simulink model "example2"  (R2013b)
settings: Solver=ode3  StartTime=0.0  StopTime=60  FixedStep=0.001  RelTol=1e-3
settings Model: Creator=Jin  LastModifiedBy=Jin

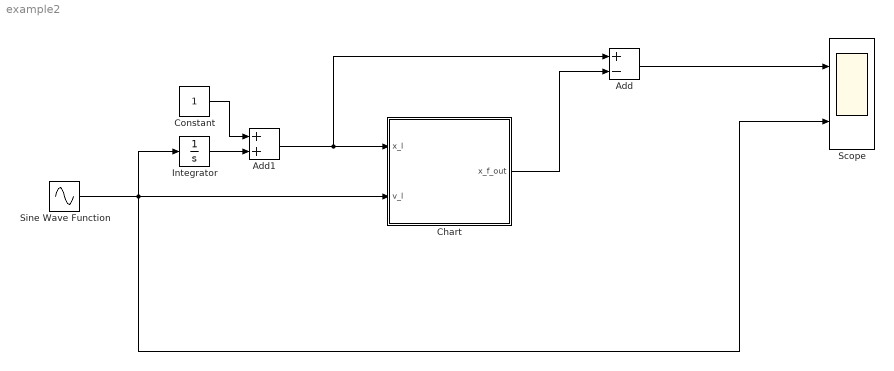
== system example2 ==
  Add : Sum  Inputs=+-
  Add1 : Sum
  Chart : Stateflow chart  TreatAsAtomicUnit=on
  Constant : Constant
  Integrator : Integrator
  Scope : Scope  NumInputPorts=2
      settings: YMin=-5~-5  YMax=5~5
  Sine Wave Function : Sin  Amplitude=5  SampleTime=0
  wires:
  Chart/1(x_f_out) -> Add/2
  Add/1 -> Scope/1
  Constant/1 -> Add1/1
  Integrator/1 -> Add1/2
  Add1/1 -> Add/1, Chart/1(x_l)
  Sine Wave Function/1 -> Scope/2, Chart/2(v_l), Integrator/1

== stateflow chart example2/Chart ==
  settings: updateMethod=CONTINUOUS
  state Drive
    du:
    x_f_dot = -6 + pow(12 * (x_l - x_f - 2 + pow(v_l,2) / 12 ) + 36, 0.5) ;
    x_f_out = x_l - x_f;
  state Collision
    du:
    x_f_dot = 0;
    x_f_out = x_l - x_f;
  (default) -> Drive : {x_f = 0;}
  Drive -> Collision : [x_l - x_f == 0]
  data: x_f local double; x_f_out output double; x_l input double; v_l input
  data x_f settings: updateMethod=SF_CONTINUOUS_TIME_DATA
